simulink model "maglevClosedLoop"  (R2024b)
settings: Solver=VariableStepAuto  StartTime=0.0  StopTime=10  FixedStep=1e-3  MaxStep=0.005  RelTol=1e-3  AbsTol=1e-5
model workspace (MATLAB code in the model file):
  | Ts=1e-3;
values from neighbouring files (symbols this model uses):
  alpha = 1.241578125e-3*m    (= 2.48315625e-05)    [MaglevDesign.m]
  g = 9.81    [MaglevDesign.m]
  gamma = 143.48    [MaglevDesign.m]
  h0 = s0    (= 0.022)    [MaglevDesign.m]
  hdot0 = 0    [MaglevDesign.m]
  kd = -0.029    [MaglevDesign.m]
  ki = -1.6    [MaglevDesign.m]
  kp = -2.15    [MaglevDesign.m]
  m = 20e-3    (= 0.02)    [MaglevDesign.m]
  NoiseVariance = 5e-5    (= 5e-05)    [MaglevDesign.m]
  s0 = 0.022    [MaglevDesign.m]
  StepTime = 5    [MaglevDesign.m]
  StepValue = 0.004*gamma    (= 0.57392)    [MaglevDesign.m]
  umax = 5    [MaglevDesign.m]
  umin = -5    [MaglevDesign.m]
Description:
  | Magnetic Levitation Model
  | 
  | vrmaglev is an example showing the interaction between dynamic models in Simulink(R)
  | and virtual worlds. The Simulink model represents the HUMUSOFT(R) CE152 Magnetic Levitation
  | educational / presentation scale model. (http://www.humusoft.com/link/models)
  | 
  | The plant model is controlled by a PID controller with feed forward to cope with the nonlinearity
  | of the magnetic levitation system.
  | 
  | The position of the ball responds to the changing value of the setpoint. You can observe
  | this change not only in the Scope window, but also in a viewer window displaying
  | the virtual world. Note that the position of the ball represents the real dynamics of the system.
  | If you switch the VRML viewer to the Camera 3 viewpoint, you can observe and control the ball easier.
  | 
  | There are two possible methods of setting the ball position setpoint - using a Signal Generator
  | and visually by clicking at a desired position in the virtual reality scene.
  | 
  | In the virtual scene, a VRML sensor is defined. If you click in the space between the magnetic coil
  | and the bottom plate, VRML sensor is updated and its value is read into Simulink model using the
  | VR Source block.
settings Model: ExtModeTrigDuration=5000  ExtModeTrigLevel=0.500000  Creator=The MathWorks, Inc.  LastModifiedBy=Admin
settings SolverCC: AutoScaleAbsTol=off  AlgebraicLoopSolver=TrustRegion
settings DataIOCC: SaveFormat=Array  SaveOutput=off  SaveTime=off  ReturnWorkspaceOutputs=off  SignalLoggingName=logsOut
settings OptimizationCC: BlockReduction=off  BooleanDataType=off  OptimizeBlockIOStorage=off  BufferReuse=off  GlobalBufferReuse=off  ExpressionFolding=off  ExpressionDepthLimit=2147483647  LocalBlockOutputs=off  InitFltsAndDblsToZero=on  LifeSpan=inf  OptimizeDataStoreBuffers=off  BusAssignmentInplaceUpdate=off
settings DebuggingCC: UnderspecifiedInitializationDetection=Classic  MergeDetectMultiDrivingBlocksExec=none  CheckExecutionContextPreStartOutputMsg=on  SignalResolutionControl=TryResolveAllWithWarning  MultiTaskDSMMsg=warning  MultiTaskCondExecSysMsg=none  FcnCallInpInsideContextMsg=warning  UnconnectedInputMsg=warning  UnconnectedOutputMsg=warning  UnconnectedLineMsg=warning  StateNameClashWarn=warning  SymbolicDimsDataTypeCodeGenerationDiagnostic=none  SFUnexpectedBacktrackingDiag=warning  SFNoUnconditionalDefaultTransitionDiag=warning  SFExecutionAtInitializationDiag=none  ArithmeticOperatorsInVariantConditions=warning
settings HardwareCC: ProdBitPerPointer=32  ProdBitPerSizeT=32  ProdBitPerPtrDiffT=32  ProdLargestAtomicFloat=None  ProdIntDivRoundTo=Undefined  ProdEndianess=Unspecified  ProdWordSize=32  ProdHWDeviceType=32-bit Generic  TargetUnknown=on
settings ModelReferenceCC: UpdateModelReferenceTargets=IfOutOfDate  EnableRefExpFcnMdlSchedulingChecks=on  PropagateSignalLabelsOutOfModel=off
settings SFSimCC: SimUseLocalCustomCode=off  CustomCodeUndefinedFunction=UseInterfaceOnly
settings RTWCC: RetainRTWFile=on  RTWUseLocalCustomCode=off  GPUComputeCapability=3.5  DLArmComputeVersion=19.05
settings CodeAppCC: StateflowObjectComments=on
settings GRTTargetCC: TargetFcnLib=ansi_tfl_tmw.mat  TargetLangStandard=C89/C90 (ANSI)  CombineOutputUpdateFcns=off  GRTInterface=on
settings ConfigComp: CovMetricSettings=d  CovSaveCumulativeToWorkspaceVar=on  CovSaveSingleToWorkspaceVar=on  CovExternalEMLEnable=off  CovSFcnEnable=off

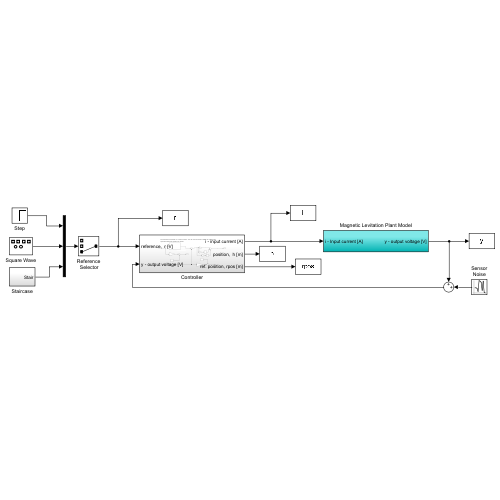
[thumbnail: Simulink's stored preview of the top-level diagram]
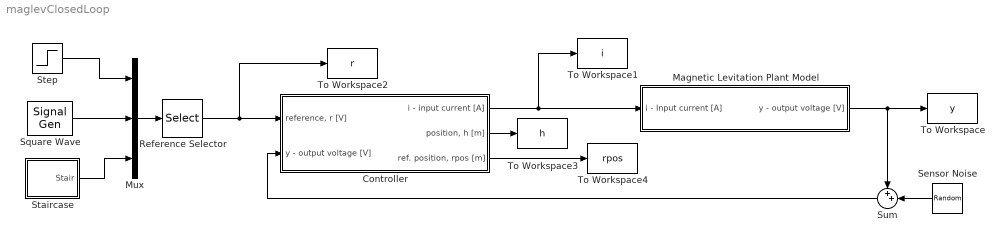
== system maglevClosedLoop ==
  Controller : Subsystem
  Magnetic Levitation Plant Model : Subsystem
  Mux : Mux  Inputs=3
  Reference Selector : Selector  InputPortWidth=3  IndexOptions=Index vector (dialog)  Indices=RefSignal  OutputSizes=1
  Sensor Noise : RandomNumber  Variance=NoiseVariance  SampleTime=0.01
  Square Wave : SignalGenerator  WaveForm=square  Amplitude=0.006*gamma  Frequency=1/8
  Staircase : Subsystem
  Step : Step  Time=StepTime  After=StepValue  SampleTime=0
  Sum : Sum  Inputs=++|
  To Workspace : ToWorkspace  VariableName=y  SaveFormat=Timeseries  SampleTime=-1
  To Workspace1 : ToWorkspace  VariableName=i  SaveFormat=Timeseries  SampleTime=-1
  To Workspace2 : ToWorkspace  VariableName=r  SaveFormat=Timeseries  SampleTime=-1
  To Workspace3 : ToWorkspace  VariableName=h  SaveFormat=Timeseries  SampleTime=-1
  To Workspace4 : ToWorkspace  VariableName=rpos  SaveFormat=Timeseries  SampleTime=-1
  wires:
  Magnetic Levitation Plant Model/1(y - output voltage [V]) -> Sum/1, To Workspace/1
  Sum/1 -> Controller/2(y - output voltage [V])
  Sensor Noise/1 -> Sum/2
  Controller/1(i - input current [A]) -> To Workspace1/1, Magnetic Levitation Plant Model/1(i - Input current [A])
  Controller/2("position, h [m]") -> To Workspace3/1
  Reference Selector/1 -> To Workspace2/1, Controller/1("reference, r [V]")
  Mux/1 -> Reference Selector/1
  Staircase/1(Stair) -> Mux/3
  Step/1 -> Mux/1
  Square Wave/1 -> Mux/2
  Controller/3("ref. position, rpos [m]") -> To Workspace4/1

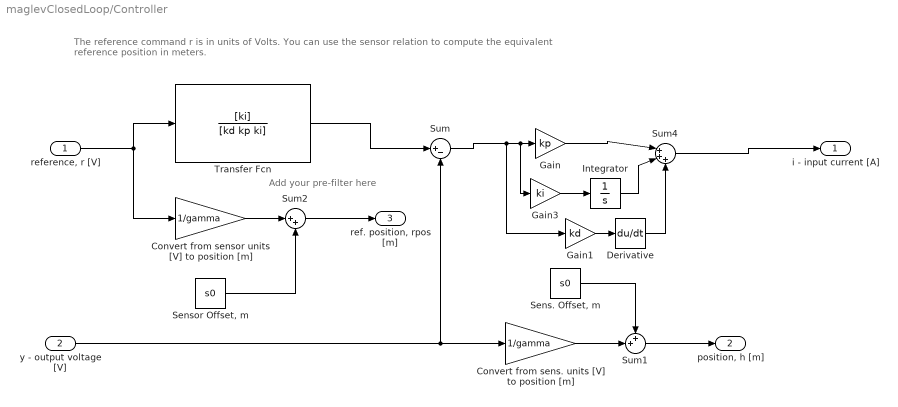
== system maglevClosedLoop/Controller ==
  note: Add your pre-filter here
  note: The reference command r is in units of Volts. You can use the sensor relation to compute the
      | equivalent reference position in meters.
  "reference, r [V]" : Inport
  y - output voltage [V] : Inport  Port=2
  Convert from sens. units [V] to position [m] : Gain  Gain=1/gamma  SaturateOnIntegerOverflow=on  OutDataTypeStr=Inherit: Same as input  ParamDataTypeStr=Inherit: Same as input
  Convert from sensor units [V] to position [m] : Gain  Gain=1/gamma  SaturateOnIntegerOverflow=on  OutDataTypeStr=Inherit: Same as input  ParamDataTypeStr=Inherit: Same as input
  Derivative : Derivative
  Gain : Gain  Gain=kp
  Gain1 : Gain  Gain=kd
  Gain3 : Gain  Gain=ki
  Integrator : Integrator
  "Sens. Offset, m" : Constant  Value=s0
  "Sensor Offset, m" : Constant  Value=s0
  Sum : Sum  Inputs=|+-  InputSameDT=on  SaturateOnIntegerOverflow=on  OutDataTypeStr=Inherit: Same as first input
  Sum1 : Sum  Inputs=++|  InputSameDT=on  SaturateOnIntegerOverflow=on  OutDataTypeStr=Inherit: Same as first input
  Sum2 : Sum  Inputs=|++  InputSameDT=on  SaturateOnIntegerOverflow=on  OutDataTypeStr=Inherit: Same as first input
  Sum4 : Sum  Inputs=|+++
  Transfer Fcn : TransferFcn  Numerator=[ki]  Denominator=[kd kp ki]
  i - input current [A] : Outport
  "position, h [m]" : Outport  Port=2
  "ref. position, rpos [m]" : Outport  Port=3
  wires:
  "reference, r [V]"/1 -> Transfer Fcn/1, Convert from sensor units [V] to position [m]/1
  y - output voltage [V]/1 -> Sum/2, Convert from sens. units [V] to position [m]/1
  Sum1/1 -> "position, h [m]"/1
  Sum2/1 -> "ref. position, rpos [m]"/1
  Convert from sensor units [V] to position [m]/1 -> Sum2/1
  Convert from sens. units [V] to position [m]/1 -> Sum1/2
  "Sens. Offset, m"/1 -> Sum1/1
  "Sensor Offset, m"/1 -> Sum2/2
  Gain1/1 -> Derivative/1
  Gain/1 -> Sum4/1
  Gain3/1 -> Integrator/1
  Sum/1 -> Gain1/1, Gain3/1, Gain/1
  Integrator/1 -> Sum4/2
  Derivative/1 -> Sum4/3
  Sum4/1 -> i - input current [A]/1
  Transfer Fcn/1 -> Sum/1

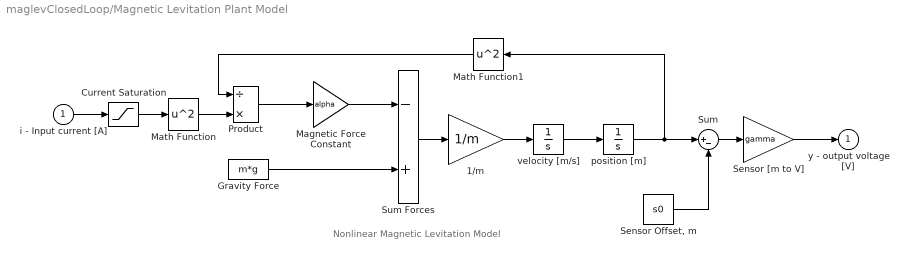
== system maglevClosedLoop/Magnetic Levitation Plant Model ==
  note: Nonlinear Magnetic
      | Levitation Model
  i - Input current [A] : Inport
  1/m : Gain  Gain=1/m  SaturateOnIntegerOverflow=on  OutDataTypeStr=Inherit: Same as input  ParamDataTypeStr=Inherit: Same as input
  Current Saturation : Saturate  UpperLimit=umax  LowerLimit=umin  ZeroCross=off
  Gravity Force : Constant  Value=m*g
  Magnetic Force Constant : Gain  Gain=alpha  SaturateOnIntegerOverflow=on  OutDataTypeStr=Inherit: Same as input  ParamDataTypeStr=Inherit: Same as input
  Math Function : Math  Operator=square  SignedPower=on
  Math Function1 : Math  Operator=square  SignedPower=on
  Product : Product  Inputs=/*  InputSameDT=on  SaturateOnIntegerOverflow=on  OutDataTypeStr=Inherit: Same as first input
  "Sensor Offset, m" : Constant  Value=s0
  Sensor [m to V] : Gain  Gain=gamma  SaturateOnIntegerOverflow=on  OutDataTypeStr=Inherit: Same as input  ParamDataTypeStr=Inherit: Same as input
  Sum : Sum  Inputs=|+-
  Sum Forces : Sum  Inputs=-+  InputSameDT=on  SaturateOnIntegerOverflow=on  OutDataTypeStr=Inherit: Same as first input
  position [m] : Integrator  InitialCondition=h0  UpperSaturationLimit=0.005  LowerSaturationLimit=0  ZeroCross=off
  velocity [m/s] : Integrator  InitialCondition=hdot0  UpperSaturationLimit=Inf  LowerSaturationLimit=-Inf  ZeroCross=off
  y - output voltage [V] : Outport  VectorParamsAs1DForOutWhenUnconnected=off
  wires:
  velocity [m/s]/1 -> position [m]/1
  1/m/1 -> velocity [m/s]/1
  Sum Forces/1 -> 1/m/1
  Gravity Force/1 -> Sum Forces/2
  position [m]/1 -> Sum/1, Math Function1/1
  Sensor [m to V]/1 -> y - output voltage [V]/1
  i - Input current [A]/1 -> Current Saturation/1
  Math Function/1 -> Product/2
  Product/1 -> Magnetic Force Constant/1
  Magnetic Force Constant/1 -> Sum Forces/1
  Current Saturation/1 -> Math Function/1
  Math Function1/1 -> Product/1
  Sum/1 -> Sensor [m to V]/1
  "Sensor Offset, m"/1 -> Sum/2

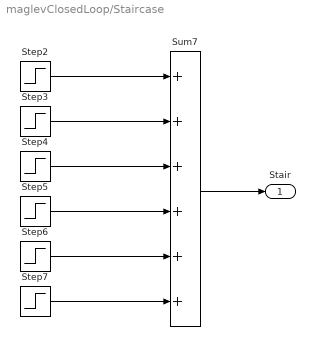
== system maglevClosedLoop/Staircase ==
  Step2 : Step  Time=10  Before=-1  After=-0.5  SampleTime=0
  Step3 : Step  Time=20  After=0.5  SampleTime=0
  Step4 : Step  Time=30  After=0.5  SampleTime=0
  Step5 : Step  Time=40  After=0.5  SampleTime=0
  Step6 : Step  Time=50  After=0.5  SampleTime=0
  Step7 : Step  Time=60  After=0.5  SampleTime=0
  Sum7 : Sum  Inputs=++++++
  Stair : Outport
  wires:
  Sum7/1 -> Stair/1
  Step2/1 -> Sum7/1
  Step3/1 -> Sum7/2
  Step4/1 -> Sum7/3
  Step5/1 -> Sum7/4
  Step6/1 -> Sum7/5
  Step7/1 -> Sum7/6
